simulink model "dual_input_disoc_v2g"  (R2020a)
settings: Solver=VariableStepAuto  StartTime=0.0  StopTime=7  RelTol=1e-3
undefined symbols (not defined in the file): Ion, Lithium, sigbuilder_block
libraries: powerlib x23, powerlib_meascontrol x12, electricdrivelib x1, re_lib x1
settings Model: Creator=Kannan Krishna  LastModifiedBy=Kannan
settings DataIOCC: ReturnWorkspaceOutputs=off
settings OptimizationCC: LifeSpan=inf
settings DebuggingCC: SFExecutionAtInitializationDiag=none  ArithmeticOperatorsInVariantConditions=warning
settings SFSimCC: SimUseLocalCustomCode=off  CustomCodeUndefinedFunction=UseInterfaceOnly
settings RTWCC: RTWUseLocalCustomCode=off
settings CodeAppCC: StateflowObjectComments=on

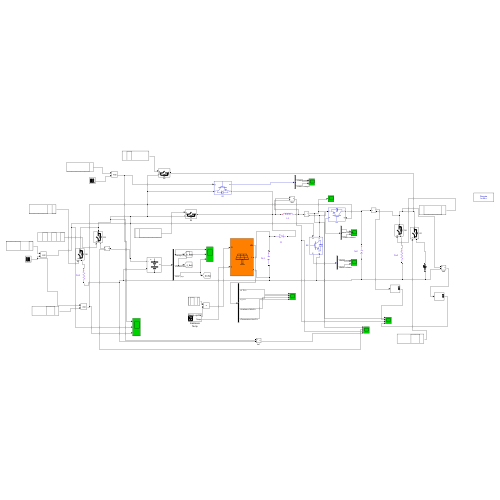
[thumbnail: Simulink's stored preview of the top-level diagram]
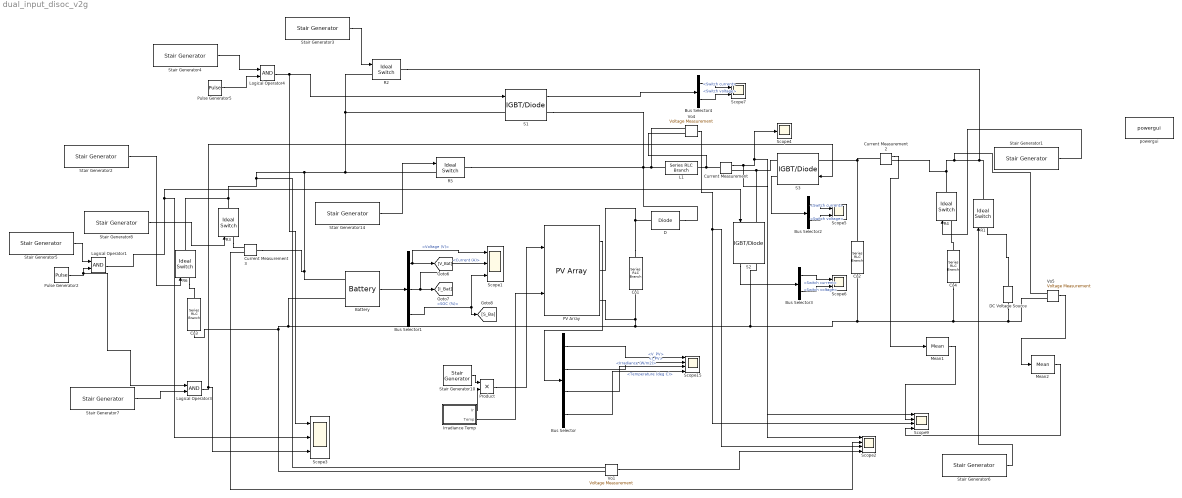
== system dual_input_disoc_v2g ==
  Battery : electricdrivelib/Extra Sources/Battery  BatType=Lithium-Ion  ShowTempParam=off  ThermalPreset=no  ShowAgeParam=off  NomV=36  NomQ=80  SOC=80  Batt_Tr=0.1  PresetModel=on  MaxQ=80  MinV=27  FullV=41.9035  Dis_rate=34.7826  R=0.0045  Normal_OP=72.3478  expZone="[38.8939      3.93043]"  current=[6.5 13 32.5]  Units=Time  Tci=20  NomT=20  T2=-30  MaxQ2=4.8  FullV2=7.1  Normal_OP2=5.655  expZone2="[6.58           1]"  Rca=0.6  ti=2000  Dp=0  Neq0=0  Tsim=1e6  Ta1=25  Qeol=5.4*0.9  Reol=0.013333*1.2  Char_age=[2.3478, 3]  Dis_age=[2.3478, 10]  N1=1500  N2=10500  N3=1000  N4=1400  Ta2=45  N5=950
  Bus Selector : BusSelector  OutputSignals=V_PV,I_PV,Irradiance (W/m2),Temperature (deg C)
  Bus Selector1 : BusSelector  OutputSignals=Voltage (V),Current (A),SOC (%)
  Bus Selector2 : BusSelector  OutputSignals=Switch current,Switch voltage
  Bus Selector3 : BusSelector  OutputSignals=Switch current,Switch voltage
  Bus Selector4 : BusSelector  OutputSignals=Switch current,Switch voltage
  Co1 : powerlib/Elements/Series RLC Branch  LConnTagsString=__new0  RConnTagsString=__new0  BranchType=C  Resistance=1  Inductance=1e-3  SetiL0=off  InitialCurrent=0  Capacitance=100E-6  Setx0=off  InitialVoltage=0  Measurements=None
  Co2 : powerlib/Elements/Series RLC Branch  LConnTagsString=__new0  RConnTagsString=__new0  BranchType=C  Resistance=1  Inductance=1e-3  SetiL0=off  InitialCurrent=0  Capacitance=470e-6  Setx0=off  InitialVoltage=0  Measurements=None
  Co3 : powerlib/Elements/Series RLC Branch  LConnTagsString=__new0  RConnTagsString=__new0  BranchType=R  Resistance=10  Inductance=1e-3  SetiL0=off  InitialCurrent=0  Capacitance=470e-6  Setx0=off  InitialVoltage=0  Measurements=None
  Co4 : powerlib/Elements/Series RLC Branch  LConnTagsString=__new0  RConnTagsString=__new0  BranchType=R  Resistance=12.5  Inductance=1e-3  SetiL0=off  InitialCurrent=0  Capacitance=470e-6  Setx0=off  InitialVoltage=0  Measurements=None
  Current Measurement : powerlib/Measurements/Current Measurement  PhasorSimulation=off  OutputType=Complex  PSBequivalent=0
  Current Measurement2 : powerlib/Measurements/Current Measurement  PhasorSimulation=off  OutputType=Complex  PSBequivalent=0
  Current Measurement3 : powerlib/Measurements/Current Measurement  PhasorSimulation=off  OutputType=Complex  PSBequivalent=0
  D : powerlib/Power Electronics/Diode  Ron=0.001  Lon=0  Vf=0.8  IC=0  UseSnubber=off  Rs=500*inf  Cs=250e-9  Measurements=off
  DC Voltage Source : powerlib/Electrical Sources/DC Voltage Source  Amplitude=48  Measurements=None
  Irradiance Temp : Subsystem  Tag=STV Subsys  LoadFcn=sigbuilder_block('load');  StartFcn=sigbuilder_block('start');  StopFcn=sigbuilder_block('stop');  ClipboardFcn=sigbuilder_block('clipboard');  mask(Sigbuilder block){tuvar=[0:10]}
      mask help: Sigbuilder GUI
      mask init:
      | if ~strcmp(get_param(bdroot(gcbh),'SimulationStatus'),'stopped') tuvar = sigbuilder_block('maskInit'); end
      settings: CopyFcn=sigbuilder_block('copy');  DeleteFcn=sigbuilder_block('delete');  ModelCloseFcn=sigbuilder_block('modelClose');  PreSaveFcn=sigbuilder_block('preSave');  PauseFcn=sigbuilder_block('pause')  ContinueFcn=sigbuilder_block('continue')  NameChangeFcn=sigbuilder_block('namechange');  OpenFcn=sigbuilder_block('open',[0 0 492.75 360.75 ]);  CloseFcn=sigbuilder_block('close');
      mask Display: plot(0, 0, 100, 100,[2, 2, 32, 32, 2], [68, 8, 8, 68, 68],[32, 2], [38, 38], [32, 19, 2],[53, 60, 44], [32, 17, 17, 2],[16, 16, 31, 31]);txt = getActiveGroup(gcbh);text(2, 100, txt,'verticalAlignment', 'top');
  L1 : powerlib/Elements/Series RLC Branch  LConnTagsString=__new0  RConnTagsString=__new0  BranchType=L  Resistance=500  Inductance=3e-3  SetiL0=off  InitialCurrent=0  Capacitance=1e-6  Setx0=off  InitialVoltage=0  Measurements=None
  Logical Operator1 : Logic  AllPortsSameDT=off  OutDataTypeStr=boolean
  Logical Operator3 : Logic  AllPortsSameDT=off  OutDataTypeStr=boolean
  Logical Operator4 : Logic  AllPortsSameDT=off  OutDataTypeStr=boolean
  Mean1 : powerlib_meascontrol/Measurements/Mean  Freq=100  Vinit=0  Ts=0
  Mean2 : powerlib_meascontrol/Measurements/Mean  Freq=100  Vinit=0  Ts=0
  PV Array : re_lib/Solar/PV Array  Npar=1  Nser=1  PlotType=one module @ 25 deg.C & specified irradiances  S_vec="[ 1000 800 500  250 ]"  Temp_C_vec="[0 25 50  ]"  ModuleName=Upsolar UP-M240M  PlotWhenSelected=on  Pm=239.3168  Ncell=60  Voc=37.53  Isc=8.5  Vm=29.84  Im=8.02  beta_Voc_pc=-0.3818  alpha_Isc_pc=-0.051  beta_Voc=-0.14329  alpha_Isc=-0.004335  IL=8.522  I0=5.1201e-10  nI=1.0347  Rsh=831.813  Rs=0.38633  RobustModel=off  RobustCellTemperature=313.3991  BAL=on  Tc=Tc  Tfilter=5e-5
  Product : Product
  Pulse Generator2 : DiscretePulseGenerator  PulseType=Time based  Period=1/20000  PulseWidth=30
  Pulse Generator5 : DiscretePulseGenerator  PulseType=Time based  Period=1/20000  PulseWidth=15
  R{1..6} (6 alike) : powerlib/Power Electronics/Ideal Switch  Ron=0.001  Lon=0  IC=0  Rs=1e5  Cs=inf  Measurements=off
  S1 : powerlib/Power Electronics/IGBT//Diode  Ron=1e-3  Rs=1e5  Cs=inf  Measurements=on
  S2 : powerlib/Power Electronics/IGBT//Diode  Ron=1e-3  Rs=1e5  Cs=inf  Measurements=on
  S3 : powerlib/Power Electronics/IGBT//Diode  Ron=1e-3  Rs=1e5  Cs=inf  Measurements=on
  Scope1 : Scope  NumInputPorts=3
  Scope15 : Scope  NumInputPorts=4
  Scope2 : Scope  NumInputPorts=4
  Scope3 : Scope  NumInputPorts=3
  Scope4 : Scope
  Scope5 : Scope  NumInputPorts=2
  Scope6 : Scope  NumInputPorts=2
  Scope7 : Scope  NumInputPorts=2
  Scope9 : Scope  NumInputPorts=4
  Stair Generator1 : powerlib_meascontrol/Pulse & Signal Generators/Stair Generator  t=[0,1,1.1, 2,2.1,3,3.1,4,4.1,5,5.1,6,6.1,7]  e=[1,1,1,1,0,0,0,0,0,0,0,0,1,1]  Ts=0
  Stair Generator10 : powerlib_meascontrol/Pulse & Signal Generators/Stair Generator  t=[0,1,1.1, 2,2.1,3,3.1,4,4.1,5,5.1,6,6.1,7]  e=[1,1,0,0,1,1,1,1,0,0,0,0,1,1]  Ts=0
  Stair Generator14 : powerlib_meascontrol/Pulse & Signal Generators/Stair Generator  t=[0,1,1.1, 2,2.1,3,3.1,4,4.1,5,5.1,6,6.1,7]  e=[0,0,1,1,0,0,0,0,0,0,0,0,0,0]  Ts=0
  Stair Generator2 : powerlib_meascontrol/Pulse & Signal Generators/Stair Generator  t=[0,1,1.1, 2,2.1,3,3.1,4,4.1,5,5.1,6,6.1,7]  e=[0,0,0,0,0,0,0,0,0,0,1,1,0,0]  Ts=0
  Stair Generator3 : powerlib_meascontrol/Pulse & Signal Generators/Stair Generator  t=[0,1,1.1, 2,2.1,3,3.1,4,4.1,5,5.1,6,6.1,7]  e=[0,0,0,0,1,1,0,0,0,0,0,0,0,0]  Ts=0
  Stair Generator4 : powerlib_meascontrol/Pulse & Signal Generators/Stair Generator  t=[0,1,1.1, 2,2.1,3,3.1,4,4.1,5,5.1,6,6.1,7]  e=[0,0,0,0,0,0,0,0,0,0,0,0,1,1]  Ts=0
  Stair Generator5 : powerlib_meascontrol/Pulse & Signal Generators/Stair Generator  t=[0,1,1.1, 2,2.1,3,3.1,4,4.1,5,5.1,6,6.1,7]  e=[1,1,1,1,1,1,1,1,0,0,0,0,1,1]  Ts=0
  Stair Generator6 : powerlib_meascontrol/Pulse & Signal Generators/Stair Generator  t=[0,1,1.1, 2,2.1,3,3.1,4,4.1,5,5.1,6,6.1,7]  e=[0,0,0,0,0,0,0,0,1,1,1,1,0,0]  Ts=0
  Stair Generator7 : powerlib_meascontrol/Pulse & Signal Generators/Stair Generator  t=[0,1,1.1, 2,2.1,3,3.1,4,4.1,5,5.1,6,6.1,7]  e=[0,0,0,0,0,0,0,0,1,1,1,1,0,0]  Ts=0
  Stair Generator8 : powerlib_meascontrol/Pulse & Signal Generators/Stair Generator  t=[0,1,1.1, 2,2.1,3,3.1,4,4.1,5,5.1,6,6.1,7]  e=[0,0,0,0,1,1,0,0,1,1,0,0,1,1]  Ts=0
  Vo1 : powerlib/Measurements/Voltage Measurement  PhasorSimulation=off  OutputType=Complex  PSBequivalent=0
  Vo4 : powerlib/Measurements/Voltage Measurement  PhasorSimulation=off  OutputType=Complex  PSBequivalent=0
  Vo5 : powerlib/Measurements/Voltage Measurement  PhasorSimulation=off  OutputType=Complex  PSBequivalent=0
  powergui : powerlib/powergui  Priority=1  SimulationMode=Discrete  SampleTime=1e-6  frequency=60  Iterations=50  frequencyindice=0  Pbase=100e6  ErrMax=1e-4  UnitsV=kV  UnitsW=MW  buscounter=0  FunctionMessages=off  echomessages=off  EnableUseOfTLC=off  CurrentSourceSwitches=off  DisableSnubberDevices=off  DisableRonSwitches=off  DisableVfSwitches=off  DisplayEquations=off  AutomaticDiscreteSolvers=off  SolverType=Tustin/Backward Euler (TBE)  Interpol=off  ExternalGateDelay=off  methode=off  Ts=100  x0status=blocks  SPID=off  SwTol=0  HookPort=off  NonlinearTolerance=1e-4  nMaxIteration=100  ContinueOnMaxIteration=off  RestoreLinks=warning  ResistiveCurrentMeasurement=off  Frange=[0:2:500]  Ylog=off  Xlog=on  ShowGrid=off  save=off  variable=ZData  structure=0  ZoomFFT=off  StartTime=0.0  cycles=1  DisplayStyle=1  fundamental=60  FreqAxis=off  MaxFrequency=1000  frequencyindicesteady=1  RmsSteady=1  display=off
  wires:
  Stair Generator1/1 -> R4/1
  Stair Generator5/1 -> Logical Operator1/1
  Bus Selector1/3 -> Scope1/3, [S_Ba]  "<SOC (%)>"
  Battery/1 -> Bus Selector1/1
  Bus Selector1/2 -> [I_Bat], Scope1/2  "<Current (A)>"
  Bus Selector1/1 -> [V_Bat], Scope1/1  "<Voltage (V)>"
  Pulse Generator5/1 -> Logical Operator4/2
  Stair Generator4/1 -> Logical Operator4/1
  Logical Operator4/1 -> Scope3/1, S1/1
  Logical Operator1/1 -> Scope3/2, S2/1
  Pulse Generator2/1 -> Logical Operator3/1, Logical Operator1/2
  Logical Operator3/1 -> Scope3/3, S3/1
  Stair Generator3/1 -> R2/1
  Stair Generator7/1 -> Logical Operator3/2
  Current Measurement/1 -> Scope9/1, Scope2/1, Scope4/1
  S3/1 -> Bus Selector2/1
  Bus Selector2/1 -> Scope5/1  "<Switch current>"
  Bus Selector2/2 -> Scope5/2  "<Switch voltage>"
  S2/1 -> Bus Selector3/1
  Bus Selector3/1 -> Scope6/1  "<Switch current>"
  Bus Selector3/2 -> Scope6/2  "<Switch voltage>"
  Bus Selector4/2 -> Scope7/2  "<Switch voltage>"
  Bus Selector4/1 -> Scope7/1  "<Switch current>"
  S1/1 -> Bus Selector4/1
  Vo4/1 -> Scope2/3, Scope9/3
  Stair Generator6/1 -> R1/1
  Stair Generator8/1 -> R3/1
  Current Measurement2/1 -> Mean1/1
  Current Measurement3/1 -> Scope2/2
  Stair Generator14/1 -> R5/1
  Vo1/1 -> Scope2/4
  PV Array/1 -> Bus Selector/1
  Stair Generator10/1 -> Product/1
  Bus Selector/4 -> Scope15/4  "<Temperature (deg C)>"
  Bus Selector/3 -> Scope15/3  "<Irradiance (W/m2)>"
  Irradiance Temp/1(Ir) -> Product/2
  Irradiance Temp/2(Temp) -> PV Array/2
  Bus Selector/2 -> Scope15/2  "<I_PV>"
  Product/1 -> PV Array/1
  Bus Selector/1 -> Scope15/1  "<V_PV>"
  Mean1/1 -> Scope9/2
  Vo5/1 -> Mean2/1
  Mean2/1 -> Scope9/4
  Stair Generator2/1 -> R6/1
  connections:
  PV Array/RConn2 -- Co4/RConn1 -- Vo5/LConn2 -- DC Voltage Source/LConn1 -- Co2/RConn1 -- S2/RConn1 -- Co3/RConn1 -- Vo1/LConn2 -- Battery/LConn2 -- Co1/RConn1
  R3/LConn1 -- Current Measurement3/RConn1
  R1/LConn1 -- DC Voltage Source/RConn1
  R5/LConn1 -- R6/RConn1 -- R3/RConn1 -- Vo1/LConn1 -- Current Measurement3/LConn1 -- Battery/LConn1 -- R2/LConn1 -- S1/LConn1
  S1/RConn1 -- D/RConn1 -- Vo4/LConn1 -- L1/LConn1 -- R5/RConn1
  S3/RConn1 -- Current Measurement/RConn1 -- S2/LConn1
  R1/RConn1 -- R2/RConn1 -- Vo5/LConn1 -- Current Measurement2/RConn1 -- R4/RConn1
  Current Measurement/LConn1 -- Vo4/LConn2 -- L1/RConn1
  Co2/LConn1 -- Current Measurement2/LConn1 -- S3/LConn1
  Co1/LConn1 -- PV Array/RConn1 -- D/LConn1
  R6/LConn1 -- Co3/LConn1
  Co4/LConn1 -- R4/LConn1

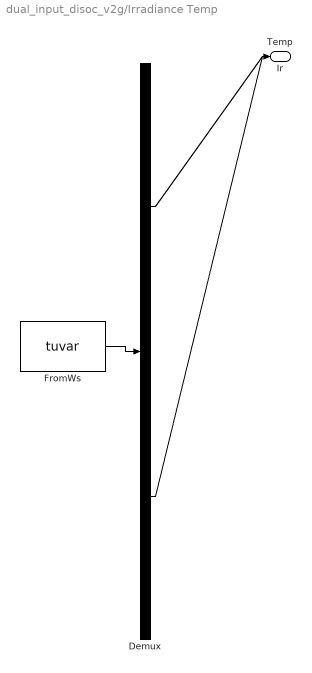
== system dual_input_disoc_v2g/Irradiance Temp ==
  Demux : Demux  Tag=STV Demux  Outputs=2
      settings: DisplayOption=none
  FromWs : FromWorkspace  Tag=STV FromWs  VariableName=tuvar
      SigBuilderData=|
      | common.afterFinalStr = 'Extrapolate'
      | common.sampleTime = '0'
      | dataSet(1).timeRange = [0 2]
      | dataSet(1).name = 'Constant Irradiance'
      | dataSet(2).timeRange = [0 4]
      | dataSet(2).name = 'Step Irradiance'
      | dataSet(3).timeRange = [0 2]
      | dataSet(3).name = 'Ramp-up/down Irradiance'
      | sbobj.Groups(1).Name = 'Constant Irradiance'
      | sbobj.Groups(1).Signals(1).Name = 'Ir'
      | sbobj.Groups(1).Signals(1).XData = [0 2]
      | sbobj.Groups(1).Signals(1).YData = [1000 1000]
      | sbobj.Groups(1).Signals(2).Name = 'Temp'
      | sbobj.Groups(1).Signals(2).XData = [0 1 1 2]
      | sbobj.Groups(1).Signals(2).YData = [0 0 1 1]
      | sbobj.Groups(1).TimeRange = [0 2]
      | sbobj.Groups(2).Name = 'Step Irradiance'
      | sbobj.Groups(2).Signals(1).Name = 'Ir'
      | sbobj.Groups(2).Signals(1).XData = [0 1 1 4]
      | sbobj.Groups(2).Signals(1).YData = [1000 1000 800 800]
      | sbobj.Groups(2).Signals(2).Name = 'Temp'
      | sbobj.Groups(2).Signals(2).XData = [0 1 1 4]
      | sbobj.Groups(2).Signals(2).YData = [0 0 1 1]
      | sbobj.Groups(2).TimeRange = [0 4]
      | sbobj.Groups(3).Name = 'Ramp-up/down Irradiance'
      | sbobj.Groups(3).Signals(1).Name = 'Ir'
      | sbobj.Groups(3).Signals(1).XData = [0 1 2]
      | sbobj.Groups(3).Signals(1).YData = [980 980 980]
      | sbobj.Groups(3).Signals(2).Name = 'Temp'
      | sbobj.Groups(3).Signals(2).XData = [0 2]
      | sbobj.Groups(3).Signals(2).YData = [25 25]
      | sbobj.Groups(3).TimeRange = [0 2]
  Ir : Outport  Tag=STV Outport  VectorParamsAs1DForOutWhenUnconnected=off
  Temp : Outport  Tag=STV Outport  Port=2  VectorParamsAs1DForOutWhenUnconnected=off
  wires:
  FromWs/1 -> Demux/1
  Demux/1 -> Ir/1
  Demux/2 -> Temp/1
